simulink model "Control_try_final_2020b"  (R2020b)
settings: Solver=VariableStepAuto  StartTime=0.0  StopTime=inf  RelTol=1e-3
undefined symbols (not defined in the file or in its folder): DiscIntNeverNeededParam
libraries: mobileRoboticsLib x25
(part 4 of 7)

== system Control_try_final_2020b/Team_1_behaviour/T1R2 (attacker 1)/Team 1 Behaviour1/Subsystem1 ==
  Action Port : Inport
  In2 : Inport  Port=2
  Action Port1 : Inport  Port=3
  Constant1 : Constant  Value=5.5
  If Action Subsystem : Subsystem  TreatAsAtomicUnit=on
  If Action Subsystem1 : Subsystem  TreatAsAtomicUnit=on
  Merge : Merge
  Bx : Outport
  wires:
  Constant1/1 -> If Action Subsystem/1(In1)
  If Action Subsystem/1(reset_pos) -> Merge/1
  Action Port1/1 -> If Action Subsystem1/Action
  If Action Subsystem1/1(reset_pos) -> Merge/2
  In2/1 -> If Action Subsystem1/1(In1)
  Merge/1 -> Bx/1
  Action Port/1 -> If Action Subsystem/Action

== system Control_try_final_2020b/Team_1_behaviour/T1R2 (attacker 1)/Team 1 Behaviour1/kick_direction1 ==
  In1 : Inport
  kick : Inport  Port=2
  dF : Inport  Port=3
  Angle Finder1 : Subsystem
  Chart1 : Stateflow chart  TreatAsAtomicUnit=on
  Chart2 : Stateflow chart  TreatAsAtomicUnit=on
  Constant2 : Constant
  Cos : Trigonometry  Operator=cos
  Demux2 : Demux  Outputs=2
  Product : Product  Inputs=3
  Product1 : Product  Inputs=3
  Sin : Trigonometry
  Vector Concatenate : Concatenate  NumInputs=4
  XYZK : Outport
  wires:
  Demux2/2 -> Chart2/1(y)
  Demux2/1 -> Chart1/1(x)
  In1/1 -> Angle Finder1/1(In1), Demux2/1
  Chart1/1(Vx) -> Product/2
  Cos/1 -> Product/3
  Angle Finder1/1(angle) -> Cos/1, Sin/1
  dF/1 -> Product/1, Product1/3
  Chart2/1(Vy) -> Product1/2
  Sin/1 -> Product1/1
  Product/1 -> Vector Concatenate/1
  Product1/1 -> Vector Concatenate/2
  Constant2/1 -> Vector Concatenate/3
  kick/1 -> Vector Concatenate/4
  Vector Concatenate/1 -> XYZK/1

== system Control_try_final_2020b/Team_1_behaviour/T1R2 (attacker 1)/Team 1 Behaviour1/min_Distance_Finder ==
  R_2_sen : Inport
  R_2_loc : Inport  Port=2
  R_1_loc : Inport  Port=3
  R_3_loc : Inport  Port=4
  R_4_loc : Inport  Port=5
  Display : Display
  Display1 : Display
  Display2 : Display
  Distance1 : Subsystem
  Distance2 : Subsystem
  MATLAB Function : MATLAB Function  TreatAsAtomicUnit=on
  Min : MinMax  Inputs=2
  Min1 : MinMax  Inputs=3
  R2_O_dist_val : Subsystem
  R3_O_dist_val : Subsystem
  R4_O_dist_val : Subsystem
  zero_padding : MATLAB Function  TreatAsAtomicUnit=on
  nearest_team : Outport
  nearest_opponent : Outport  Port=2
  nearest_team_idx : Outport  Port=3
  wires:
  R_1_loc/1 -> R2_O_dist_val/2(R_2_loc)
  R_2_loc/1 -> R4_O_dist_val/1(R_1_loc), R3_O_dist_val/1(R_1_loc), R2_O_dist_val/1(R_1_loc), Distance2/1(R_1_loc), Distance1/1(R_1_loc)
  R_3_loc/1 -> R3_O_dist_val/2(R_2_loc), Distance1/2(R_3_loc)
  R_4_loc/1 -> R4_O_dist_val/2(R_2_loc), Distance2/2(R_4_loc)
  R_2_sen/1 -> zero_padding/1(u)
  zero_padding/1(y) -> R3_O_dist_val/3(sen_1_val), R4_O_dist_val/3(sen_1_val), R2_O_dist_val/3(sen_1_val)
  R2_O_dist_val/1(y) -> Min1/1, Display/1
  R3_O_dist_val/1(y) -> Min1/2, Display1/1
  R4_O_dist_val/1(y) -> Min1/3, Display2/1
  Min/1 -> MATLAB Function/1(min), nearest_team/1
  Min1/1 -> nearest_opponent/1
  Distance1/1(R1_R3_dis) -> MATLAB Function/2(rob3), Min/1
  Distance2/1(R1_R4_dis) -> Min/2
  MATLAB Function/1(y) -> nearest_team_idx/1

== system Control_try_final_2020b/Team_1_behaviour/T1R3 (Defender 2)/Team 1 Behaviour1/Angle Finder1 ==
  In1 : Inport
  Abs : Abs
  Atan : Trigonometry  Operator=atan
  Demux : Demux  Outputs=2
  Divide : Product  Inputs=/*
  angle : Outport
  wires:
  Divide/1 -> Atan/1
  Demux/2 -> Divide/2
  Demux/1 -> Divide/1
  Atan/1 -> Abs/1
  Abs/1 -> angle/1
  In1/1 -> Demux/1

== system Control_try_final_2020b/Team_1_behaviour/T1R3 (Defender 2)/Team 1 Behaviour1/Proximity_Finder_Ball1 ==
  In1 : Inport
  Demux : Demux  Outputs=2
  Sqrt : Sqrt  SaturateOnIntegerOverflow=on
  Square : Math  Operator=square  SaturateOnIntegerOverflow=on
  Square1 : Math  Operator=square  SaturateOnIntegerOverflow=on
  Sum : Sum
  DBR : Outport
  wires:
  In1/1 -> Demux/1
  Demux/1 -> Square/1
  Demux/2 -> Square1/1
  Square1/1 -> Sum/2
  Square/1 -> Sum/1
  Sum/1 -> Sqrt/1
  Sqrt/1 -> DBR/1

== system Control_try_final_2020b/Team_1_behaviour/T1R3 (Defender 2)/Team 1 Behaviour1/Proximity_Finder_Ball2 ==
  In1 : Inport
  Demux : Demux  Outputs=2
  Sqrt : Sqrt  SaturateOnIntegerOverflow=on
  Square : Math  Operator=square  SaturateOnIntegerOverflow=on
  Square1 : Math  Operator=square  SaturateOnIntegerOverflow=on
  Sum : Sum
  DBR : Outport
  wires:
  Sqrt/1 -> DBR/1
  Sum/1 -> Sqrt/1
  Square/1 -> Sum/1
  Square1/1 -> Sum/2
  Demux/2 -> Square1/1
  Demux/1 -> Square/1
  In1/1 -> Demux/1

== system Control_try_final_2020b/Team_1_behaviour/T1R3 (Defender 2)/Team 1 Behaviour1/Simulink Function ==
  f : TriggerPort  TriggerType=function-call  IsSimulinkFunction=on  FunctionName=f  FunctionVisibility=scoped  VariantControl=(inherit)
  Demux : Demux  Outputs=2
  Sqrt : Sqrt  SaturateOnIntegerOverflow=on
  Square : Math  Operator=square  SaturateOnIntegerOverflow=on
  Square1 : Math  Operator=square  SaturateOnIntegerOverflow=on
  Sum : Sum
  u : ArgIn  DisableCoverage=on  PortDimensions=[1 2]  ArgumentName=u
  y : ArgOut  DisableCoverage=on  ArgumentName=y
  wires:
  u/1 -> Demux/1
  Square/1 -> Sum/1
  Sum/1 -> Sqrt/1
  Sqrt/1 -> y/1
  Square1/1 -> Sum/2
  Demux/1 -> Square/1
  Demux/2 -> Square1/1

== system Control_try_final_2020b/Team_1_behaviour/T1R3 (Defender 2)/Team 1 Behaviour1/Subsystem1 ==
  Action Port : Inport
  In2 : Inport  Port=2
  Action Port1 : Inport  Port=3
  Constant1 : Constant  Value=3.5
  If Action Subsystem : Subsystem  TreatAsAtomicUnit=on
  If Action Subsystem1 : Subsystem  TreatAsAtomicUnit=on
  Merge : Merge
  Bx : Outport
  wires:
  Constant1/1 -> If Action Subsystem/1(In1)
  If Action Subsystem/1(reset_pos) -> Merge/1
  Action Port1/1 -> If Action Subsystem1/Action
  If Action Subsystem1/1(reset_pos) -> Merge/2
  In2/1 -> If Action Subsystem1/1(In1)
  Merge/1 -> Bx/1
  Action Port/1 -> If Action Subsystem/Action

== system Control_try_final_2020b/Team_1_behaviour/T1R3 (Defender 2)/Team 1 Behaviour1/Subsystem2 ==
  Action Port : Inport
  In2 : Inport  Port=2
  Action Port1 : Inport  Port=3
  Constant1 : Constant  Value=5.5
  If Action Subsystem : Subsystem  TreatAsAtomicUnit=on
  If Action Subsystem1 : Subsystem  TreatAsAtomicUnit=on
  Merge : Merge
  By : Outport
  wires:
  Action Port/1 -> If Action Subsystem/Action
  Merge/1 -> By/1
  In2/1 -> If Action Subsystem1/1(In1)
  If Action Subsystem1/1(reset_pos) -> Merge/2
  Action Port1/1 -> If Action Subsystem1/Action
  If Action Subsystem/1(reset_pos) -> Merge/1
  Constant1/1 -> If Action Subsystem/1(In1)

== system Control_try_final_2020b/Team_1_behaviour/T1R3 (Defender 2)/Team 1 Behaviour1/kick_direction1 ==
  In1 : Inport
  kick : Inport  Port=2
  dF : Inport  Port=3
  Angle Finder1 : Subsystem
  Chart1 : Stateflow chart  TreatAsAtomicUnit=on
  Chart2 : Stateflow chart  TreatAsAtomicUnit=on
  Constant2 : Constant
  Cos : Trigonometry  Operator=cos
  Demux2 : Demux  Outputs=2
  Product : Product  Inputs=3
  Product1 : Product  Inputs=3
  Sin : Trigonometry
  Vector Concatenate : Concatenate  NumInputs=4
  XYZK : Outport
  wires:
  Demux2/2 -> Chart2/1(y)
  Demux2/1 -> Chart1/1(x)
  In1/1 -> Angle Finder1/1(In1), Demux2/1
  Chart1/1(Vx) -> Product/2
  Cos/1 -> Product/3
  Angle Finder1/1(angle) -> Cos/1, Sin/1
  dF/1 -> Product/1, Product1/3
  Chart2/1(Vy) -> Product1/2
  Sin/1 -> Product1/1
  Product/1 -> Vector Concatenate/1
  Product1/1 -> Vector Concatenate/2
  Constant2/1 -> Vector Concatenate/3
  kick/1 -> Vector Concatenate/4
  Vector Concatenate/1 -> XYZK/1

== system Control_try_final_2020b/Team_1_behaviour/T1R3 (Defender 2)/Team 1 Behaviour1/min_Distance_Finder ==
  R_2_sen : Inport
  R_2_loc : Inport  Port=2
  R_1_loc : Inport  Port=3
  R_3_loc : Inport  Port=4
  R_4_loc : Inport  Port=5
  Display : Display
  Display1 : Display
  Display2 : Display
  Distance1 : Subsystem
  Distance2 : Subsystem
  MATLAB Function : MATLAB Function  TreatAsAtomicUnit=on
  Min : MinMax  Inputs=2
  Min1 : MinMax  Inputs=3
  R2_O_dist_val : Subsystem
  R3_O_dist_val : Subsystem
  R4_O_dist_val : Subsystem
  zero_padding : MATLAB Function  TreatAsAtomicUnit=on
  nearest_team : Outport
  nearest_opponent : Outport  Port=2
  nearest_team_idx : Outport  Port=3
  wires:
  R_1_loc/1 -> R2_O_dist_val/2(R_2_loc)
  R_2_loc/1 -> R4_O_dist_val/1(R_1_loc), R3_O_dist_val/1(R_1_loc), R2_O_dist_val/1(R_1_loc), Distance2/1(R_1_loc), Distance1/1(R_1_loc)
  R_3_loc/1 -> R3_O_dist_val/2(R_2_loc), Distance1/2(R_3_loc)
  R_4_loc/1 -> R4_O_dist_val/2(R_2_loc), Distance2/2(R_4_loc)
  R_2_sen/1 -> zero_padding/1(u)
  zero_padding/1(y) -> R3_O_dist_val/3(sen_1_val), R4_O_dist_val/3(sen_1_val), R2_O_dist_val/3(sen_1_val)
  R2_O_dist_val/1(y) -> Min1/1, Display/1
  R3_O_dist_val/1(y) -> Min1/2, Display1/1
  R4_O_dist_val/1(y) -> Min1/3, Display2/1
  Min/1 -> MATLAB Function/1(min), nearest_team/1
  Min1/1 -> nearest_opponent/1
  Distance1/1(R1_R3_dis) -> MATLAB Function/2(rob3), Min/1
  Distance2/1(R1_R4_dis) -> Min/2
  MATLAB Function/1(y) -> nearest_team_idx/1

== system Control_try_final_2020b/Team_1_behaviour/T1R3 (defender 1)/Team 1 Behaviour/Angle Finder ==
  In1 : Inport
  Abs : Abs
  Atan : Trigonometry  Operator=atan
  Demux : Demux  Outputs=2
  Divide : Product  Inputs=/*
  angle : Outport
  wires:
  Divide/1 -> Atan/1
  Demux/2 -> Divide/2
  Demux/1 -> Divide/1
  Atan/1 -> Abs/1
  Abs/1 -> angle/1
  In1/1 -> Demux/1

== system Control_try_final_2020b/Team_1_behaviour/T1R3 (defender 1)/Team 1 Behaviour/Proximity_Finder_Ball ==
  In1 : Inport
  Demux : Demux  Outputs=2
  Sqrt : Sqrt  SaturateOnIntegerOverflow=on
  Square : Math  Operator=square  SaturateOnIntegerOverflow=on
  Square1 : Math  Operator=square  SaturateOnIntegerOverflow=on
  Sum : Sum
  DBR : Outport
  wires:
  In1/1 -> Demux/1
  Demux/1 -> Square/1
  Demux/2 -> Square1/1
  Square1/1 -> Sum/2
  Square/1 -> Sum/1
  Sum/1 -> Sqrt/1
  Sqrt/1 -> DBR/1

== system Control_try_final_2020b/Team_1_behaviour/T1R3 (defender 1)/Team 1 Behaviour/kick_direction ==
  In1 : Inport
  kick : Inport  Port=2
  Angle Finder1 : Subsystem
  Chart1 : Stateflow chart  TreatAsAtomicUnit=on
  Chart2 : Stateflow chart  TreatAsAtomicUnit=on
  Constant : Constant  Value=2.5
  Constant1 : Constant  Value=2.5
  Constant2 : Constant
  Cos : Trigonometry  Operator=cos
  Demux2 : Demux  Outputs=2
  Product : Product  Inputs=3
  Product1 : Product  Inputs=3
  Sin : Trigonometry
  Vector Concatenate : Concatenate  NumInputs=4
  Out1 : Outport
  wires:
  Demux2/2 -> Chart2/1(y)
  Demux2/1 -> Chart1/1(x)
  In1/1 -> Angle Finder1/1(In1), Demux2/1
  Chart1/1(Vx) -> Product/2
  Cos/1 -> Product/3
  Angle Finder1/1(angle) -> Cos/1, Sin/1
  Constant/1 -> Product/1
  Constant1/1 -> Product1/3
  Chart2/1(Vy) -> Product1/2
  Sin/1 -> Product1/1
  Product/1 -> Vector Concatenate/1
  Product1/1 -> Vector Concatenate/2
  Constant2/1 -> Vector Concatenate/3
  kick/1 -> Vector Concatenate/4
  Vector Concatenate/1 -> Out1/1

== system Control_try_final_2020b/Team_1_behaviour/T1R3 (defender 1)/Team 1 Behaviour1/Angle Finder1 ==
  In1 : Inport
  Abs : Abs
  Atan : Trigonometry  Operator=atan
  Demux : Demux  Outputs=2
  Divide : Product  Inputs=/*
  angle : Outport
  wires:
  Divide/1 -> Atan/1
  Demux/2 -> Divide/2
  Demux/1 -> Divide/1
  Atan/1 -> Abs/1
  Abs/1 -> angle/1
  In1/1 -> Demux/1

== system Control_try_final_2020b/Team_1_behaviour/T1R3 (defender 1)/Team 1 Behaviour1/Proximity_Finder_Ball1 ==
  In1 : Inport
  Demux : Demux  Outputs=2
  Sqrt : Sqrt  SaturateOnIntegerOverflow=on
  Square : Math  Operator=square  SaturateOnIntegerOverflow=on
  Square1 : Math  Operator=square  SaturateOnIntegerOverflow=on
  Sum : Sum
  DBR : Outport
  wires:
  In1/1 -> Demux/1
  Demux/1 -> Square/1
  Demux/2 -> Square1/1
  Square1/1 -> Sum/2
  Square/1 -> Sum/1
  Sum/1 -> Sqrt/1
  Sqrt/1 -> DBR/1

== system Control_try_final_2020b/Team_1_behaviour/T1R3 (defender 1)/Team 1 Behaviour1/Proximity_Finder_Ball2 ==
  In1 : Inport
  Demux : Demux  Outputs=2
  Sqrt : Sqrt  SaturateOnIntegerOverflow=on
  Square : Math  Operator=square  SaturateOnIntegerOverflow=on
  Square1 : Math  Operator=square  SaturateOnIntegerOverflow=on
  Sum : Sum
  DBR : Outport
  wires:
  Sqrt/1 -> DBR/1
  Sum/1 -> Sqrt/1
  Square/1 -> Sum/1
  Square1/1 -> Sum/2
  Demux/2 -> Square1/1
  Demux/1 -> Square/1
  In1/1 -> Demux/1

== system Control_try_final_2020b/Team_1_behaviour/T1R3 (defender 1)/Team 1 Behaviour1/Simulink Function ==
  f : TriggerPort  TriggerType=function-call  IsSimulinkFunction=on  FunctionName=f  FunctionVisibility=scoped  VariantControl=(inherit)
  Demux : Demux  Outputs=2
  Sqrt : Sqrt  SaturateOnIntegerOverflow=on
  Square : Math  Operator=square  SaturateOnIntegerOverflow=on
  Square1 : Math  Operator=square  SaturateOnIntegerOverflow=on
  Sum : Sum
  u : ArgIn  DisableCoverage=on  PortDimensions=[1 2]  ArgumentName=u
  y : ArgOut  DisableCoverage=on  ArgumentName=y
  wires:
  u/1 -> Demux/1
  Square/1 -> Sum/1
  Sum/1 -> Sqrt/1
  Sqrt/1 -> y/1
  Square1/1 -> Sum/2
  Demux/1 -> Square/1
  Demux/2 -> Square1/1

== system Control_try_final_2020b/Team_1_behaviour/T1R3 (defender 1)/Team 1 Behaviour1/Subsystem1 ==
  Action Port : Inport
  In2 : Inport  Port=2
  Action Port1 : Inport  Port=3
  Constant1 : Constant  Value=3.5
  If Action Subsystem : Subsystem  TreatAsAtomicUnit=on
  If Action Subsystem1 : Subsystem  TreatAsAtomicUnit=on
  Merge : Merge
  Bx : Outport
  wires:
  Constant1/1 -> If Action Subsystem/1(In1)
  If Action Subsystem/1(reset_pos) -> Merge/1
  Action Port1/1 -> If Action Subsystem1/Action
  If Action Subsystem1/1(reset_pos) -> Merge/2
  In2/1 -> If Action Subsystem1/1(In1)
  Merge/1 -> Bx/1
  Action Port/1 -> If Action Subsystem/Action

== system Control_try_final_2020b/Team_1_behaviour/T1R3 (defender 1)/Team 1 Behaviour1/Subsystem2 ==
  Action Port : Inport
  In2 : Inport  Port=2
  Action Port1 : Inport  Port=3
  Constant1 : Constant  Value=2.5
  If Action Subsystem : Subsystem  TreatAsAtomicUnit=on
  If Action Subsystem1 : Subsystem  TreatAsAtomicUnit=on
  Merge : Merge
  By : Outport
  wires:
  Action Port/1 -> If Action Subsystem/Action
  Merge/1 -> By/1
  In2/1 -> If Action Subsystem1/1(In1)
  If Action Subsystem1/1(reset_pos) -> Merge/2
  Action Port1/1 -> If Action Subsystem1/Action
  If Action Subsystem/1(reset_pos) -> Merge/1
  Constant1/1 -> If Action Subsystem/1(In1)

== system Control_try_final_2020b/Team_1_behaviour/T1R3 (defender 1)/Team 1 Behaviour1/kick_direction1 ==
  In1 : Inport
  kick : Inport  Port=2
  dF : Inport  Port=3
  Angle Finder1 : Subsystem
  Chart1 : Stateflow chart  TreatAsAtomicUnit=on
  Chart2 : Stateflow chart  TreatAsAtomicUnit=on
  Constant2 : Constant
  Cos : Trigonometry  Operator=cos
  Demux2 : Demux  Outputs=2
  Product : Product  Inputs=3
  Product1 : Product  Inputs=3
  Sin : Trigonometry
  Vector Concatenate : Concatenate  NumInputs=4
  XYZK : Outport
  wires:
  Demux2/2 -> Chart2/1(y)
  Demux2/1 -> Chart1/1(x)
  In1/1 -> Angle Finder1/1(In1), Demux2/1
  Chart1/1(Vx) -> Product/2
  Cos/1 -> Product/3
  Angle Finder1/1(angle) -> Cos/1, Sin/1
  dF/1 -> Product/1, Product1/3
  Chart2/1(Vy) -> Product1/2
  Sin/1 -> Product1/1
  Product/1 -> Vector Concatenate/1
  Product1/1 -> Vector Concatenate/2
  Constant2/1 -> Vector Concatenate/3
  kick/1 -> Vector Concatenate/4
  Vector Concatenate/1 -> XYZK/1

== system Control_try_final_2020b/Team_1_behaviour/T1R3 (defender 1)/Team 1 Behaviour1/min_Distance_Finder ==
  R_2_sen : Inport
  R_2_loc : Inport  Port=2
  R_1_loc : Inport  Port=3
  R_3_loc : Inport  Port=4
  R_4_loc : Inport  Port=5
  Display : Display
  Display1 : Display
  Display2 : Display
  Distance1 : Subsystem
  Distance2 : Subsystem
  MATLAB Function : MATLAB Function  TreatAsAtomicUnit=on
  Min : MinMax  Inputs=2
  Min1 : MinMax  Inputs=3
  R2_O_dist_val : Subsystem
  R3_O_dist_val : Subsystem
  R4_O_dist_val : Subsystem
  zero_padding : MATLAB Function  TreatAsAtomicUnit=on
  nearest_team : Outport
  nearest_opponent : Outport  Port=2
  nearest_team_idx : Outport  Port=3
  wires:
  R_1_loc/1 -> R2_O_dist_val/2(R_2_loc)
  R_2_loc/1 -> R4_O_dist_val/1(R_1_loc), R3_O_dist_val/1(R_1_loc), R2_O_dist_val/1(R_1_loc), Distance2/1(R_1_loc), Distance1/1(R_1_loc)
  R_3_loc/1 -> R3_O_dist_val/2(R_2_loc), Distance1/2(R_3_loc)
  R_4_loc/1 -> R4_O_dist_val/2(R_2_loc), Distance2/2(R_4_loc)
  R_2_sen/1 -> zero_padding/1(u)
  zero_padding/1(y) -> R3_O_dist_val/3(sen_1_val), R4_O_dist_val/3(sen_1_val), R2_O_dist_val/3(sen_1_val)
  R2_O_dist_val/1(y) -> Min1/1, Display/1
  R3_O_dist_val/1(y) -> Min1/2, Display1/1
  R4_O_dist_val/1(y) -> Min1/3, Display2/1
  Min/1 -> MATLAB Function/1(min), nearest_team/1
  Min1/1 -> nearest_opponent/1
  Distance1/1(R1_R3_dis) -> MATLAB Function/2(rob3), Min/1
  Distance2/1(R1_R4_dis) -> Min/2
  MATLAB Function/1(y) -> nearest_team_idx/1

== system Control_try_final_2020b/Team_2_Behaviour/T2_R1(Goal_Keeper)/min_Distance_Finder/Distance ==
  R_1_loc : Inport
  R_2_loc : Inport  Port=2
  Demux : Demux  Outputs=3
  Demux1 : Demux  Outputs=3
  Square : Math  Operator=square  SaturateOnIntegerOverflow=on
  Square Root : Sqrt  SaturateOnIntegerOverflow=on
  Square1 : Math  Operator=square  SaturateOnIntegerOverflow=on
  Sum : Sum  Inputs=|+-
  Sum1 : Sum  Inputs=|+-
  Sum2 : Sum  Inputs=|++
  R1_R2_dis : Outport
  wires:
  Square1/1 -> Sum2/2
  Demux/2 -> Sum1/1
  Sum2/1 -> Square Root/1
  Square/1 -> Sum2/1
  Demux/1 -> Sum/1
  Sum1/1 -> Square1/1
  Demux1/2 -> Sum1/2
  Sum/1 -> Square/1
  Demux1/1 -> Sum/2
  R_1_loc/1 -> Demux/1
  R_2_loc/1 -> Demux1/1
  Square Root/1 -> R1_R2_dis/1

== system Control_try_final_2020b/Team_2_Behaviour/T2_R1(Goal_Keeper)/min_Distance_Finder/Distance1 ==
  R_1_loc : Inport
  R_3_loc : Inport  Port=2
  Demux : Demux  Outputs=3
  Demux1 : Demux  Outputs=3
  Square : Math  Operator=square  SaturateOnIntegerOverflow=on
  Square Root : Sqrt  SaturateOnIntegerOverflow=on
  Square1 : Math  Operator=square  SaturateOnIntegerOverflow=on
  Sum : Sum  Inputs=|+-
  Sum1 : Sum  Inputs=|+-
  Sum2 : Sum  Inputs=|++
  R1_R3_dis : Outport
  wires:
  Square1/1 -> Sum2/2
  Demux/2 -> Sum1/1
  Sum2/1 -> Square Root/1
  Square/1 -> Sum2/1
  Demux/1 -> Sum/1
  Sum1/1 -> Square1/1
  Demux1/2 -> Sum1/2
  Sum/1 -> Square/1
  Demux1/1 -> Sum/2
  R_1_loc/1 -> Demux/1
  R_3_loc/1 -> Demux1/1
  Square Root/1 -> R1_R3_dis/1

== system Control_try_final_2020b/Team_2_Behaviour/T2_R1(Goal_Keeper)/min_Distance_Finder/Distance2 ==
  R_1_loc : Inport
  R_4_loc : Inport  Port=2
  Demux : Demux  Outputs=3
  Demux1 : Demux  Outputs=3
  Square : Math  Operator=square  SaturateOnIntegerOverflow=on
  Square Root : Sqrt  SaturateOnIntegerOverflow=on
  Square1 : Math  Operator=square  SaturateOnIntegerOverflow=on
  Sum : Sum  Inputs=|+-
  Sum1 : Sum  Inputs=|+-
  Sum2 : Sum  Inputs=|++
  R1_R4_dis : Outport
  wires:
  Square1/1 -> Sum2/2
  Demux/2 -> Sum1/1
  Sum2/1 -> Square Root/1
  Square/1 -> Sum2/1
  Demux/1 -> Sum/1
  Sum1/1 -> Square1/1
  Demux1/2 -> Sum1/2
  Sum/1 -> Square/1
  Demux1/1 -> Sum/2
  R_1_loc/1 -> Demux/1
  R_4_loc/1 -> Demux1/1
  Square Root/1 -> R1_R4_dis/1

== system Control_try_final_2020b/Team_2_Behaviour/T2_R1(Goal_Keeper)/min_Distance_Finder/R2_O_dist_val ==
  R_1_loc : Inport
  R_2_loc : Inport  Port=2
  sen_1_val : Inport  Port=3
  Chart : Stateflow chart  TreatAsAtomicUnit=on
  y : Outport
  wires:
  sen_1_val/1 -> Chart/2(sen_1_val)
  R_1_loc/1 -> Chart/1(R_1_loc)
  R_2_loc/1 -> Chart/3(R_2_loc)
  Chart/1(dist) -> y/1

== system Control_try_final_2020b/Team_2_Behaviour/T2_R1(Goal_Keeper)/min_Distance_Finder/R3_O_dist_val ==
  R_1_loc : Inport
  R_2_loc : Inport  Port=2
  sen_1_val : Inport  Port=3
  Chart : Stateflow chart  TreatAsAtomicUnit=on
  y : Outport
  wires:
  Chart/1(dist) -> y/1
  R_2_loc/1 -> Chart/3(R_2_loc)
  R_1_loc/1 -> Chart/1(R_1_loc)
  sen_1_val/1 -> Chart/2(sen_1_val)

== system Control_try_final_2020b/Team_2_Behaviour/T2_R1(Goal_Keeper)/min_Distance_Finder/R4_O_dist_val ==
  R_1_loc : Inport
  R_2_loc : Inport  Port=2
  sen_1_val : Inport  Port=3
  Chart : Stateflow chart  TreatAsAtomicUnit=on
  y : Outport
  wires:
  sen_1_val/1 -> Chart/2(sen_1_val)
  R_1_loc/1 -> Chart/1(R_1_loc)
  R_2_loc/1 -> Chart/3(R_2_loc)
  Chart/1(dist) -> y/1

== system Control_try_final_2020b/Team_2_Behaviour/T2_R2(defender)/Team 1 Behaviour1/Angle Finder1 ==
  In1 : Inport
  Abs : Abs
  Atan : Trigonometry  Operator=atan
  Demux : Demux  Outputs=2
  Divide : Product  Inputs=/*
  angle : Outport
  wires:
  Divide/1 -> Atan/1
  Demux/2 -> Divide/2
  Demux/1 -> Divide/1
  Atan/1 -> Abs/1
  Abs/1 -> angle/1
  In1/1 -> Demux/1

== system Control_try_final_2020b/Team_2_Behaviour/T2_R2(defender)/Team 1 Behaviour1/Proximity_Finder_Ball1 ==
  In1 : Inport
  Demux : Demux  Outputs=2
  Sqrt : Sqrt  SaturateOnIntegerOverflow=on
  Square : Math  Operator=square  SaturateOnIntegerOverflow=on
  Square1 : Math  Operator=square  SaturateOnIntegerOverflow=on
  Sum : Sum
  DBR : Outport
  wires:
  In1/1 -> Demux/1
  Demux/1 -> Square/1
  Demux/2 -> Square1/1
  Square1/1 -> Sum/2
  Square/1 -> Sum/1
  Sum/1 -> Sqrt/1
  Sqrt/1 -> DBR/1

== system Control_try_final_2020b/Team_2_Behaviour/T2_R2(defender)/Team 1 Behaviour1/Proximity_Finder_Ball2 ==
  In1 : Inport
  Demux : Demux  Outputs=2
  Sqrt : Sqrt  SaturateOnIntegerOverflow=on
  Square : Math  Operator=square  SaturateOnIntegerOverflow=on
  Square1 : Math  Operator=square  SaturateOnIntegerOverflow=on
  Sum : Sum
  DBR : Outport
  wires:
  Sqrt/1 -> DBR/1
  Sum/1 -> Sqrt/1
  Square/1 -> Sum/1
  Square1/1 -> Sum/2
  Demux/2 -> Square1/1
  Demux/1 -> Square/1
  In1/1 -> Demux/1

== system Control_try_final_2020b/Team_2_Behaviour/T2_R2(defender)/Team 1 Behaviour1/Simulink Function ==
  f : TriggerPort  TriggerType=function-call  IsSimulinkFunction=on  FunctionName=f  FunctionVisibility=scoped  VariantControl=(inherit)
  Demux : Demux  Outputs=2
  Sqrt : Sqrt  SaturateOnIntegerOverflow=on
  Square : Math  Operator=square  SaturateOnIntegerOverflow=on
  Square1 : Math  Operator=square  SaturateOnIntegerOverflow=on
  Sum : Sum
  u : ArgIn  DisableCoverage=on  PortDimensions=[1 2]  ArgumentName=u
  y : ArgOut  DisableCoverage=on  ArgumentName=y
  wires:
  u/1 -> Demux/1
  Square/1 -> Sum/1
  Sum/1 -> Sqrt/1
  Sqrt/1 -> y/1
  Square1/1 -> Sum/2
  Demux/1 -> Square/1
  Demux/2 -> Square1/1

== system Control_try_final_2020b/Team_2_Behaviour/T2_R2(defender)/Team 1 Behaviour1/Subsystem ==
  Constant5 : Constant
  Constant6 : Constant  Value=4
  IC : InitialCondition  Value=0
  If : If
  If Action Subsystem : Subsystem  TreatAsAtomicUnit=on
  If Action Subsystem1 : Subsystem  TreatAsAtomicUnit=on
  Matrix Concatenate1 : Concatenate  Mode=Multidimensional array  ConcatenateDimension=2
  Merge : Merge
  Out1 : Outport
  wires:
  [centroid] -> If Action Subsystem1/1(In1)
  [A] -> IC/1
  If/1 -> If Action Subsystem/Action
  If Action Subsystem1/1(Out1) -> Merge/2
  Matrix Concatenate1/1 -> If Action Subsystem/1(In1)
  IC/1 -> If/1
  Constant6/1 -> Matrix Concatenate1/2
  Constant5/1 -> Matrix Concatenate1/1
  If/2 -> If Action Subsystem1/Action
  If Action Subsystem/1(Out1) -> Merge/1
  Merge/1 -> Out1/1

== system Control_try_final_2020b/Team_2_Behaviour/T2_R2(defender)/Team 1 Behaviour1/Subsystem1 ==
  Action Port : Inport
  In2 : Inport  Port=2
  Action Port1 : Inport  Port=3
  Constant1 : Constant  Value=7.5
  If Action Subsystem : Subsystem  TreatAsAtomicUnit=on
  If Action Subsystem1 : Subsystem  TreatAsAtomicUnit=on
  Merge : Merge
  Out1 : Outport
  wires:
  Constant1/1 -> If Action Subsystem/1(In1)
  If Action Subsystem/1(reset_pos) -> Merge/1
  Action Port1/1 -> If Action Subsystem1/Action
  If Action Subsystem1/1(reset_pos) -> Merge/2
  In2/1 -> If Action Subsystem1/1(In1)
  Merge/1 -> Out1/1
  Action Port/1 -> If Action Subsystem/Action

== system Control_try_final_2020b/Team_2_Behaviour/T2_R2(defender)/Team 1 Behaviour1/Subsystem2 ==
  Action Port : Inport
  In2 : Inport  Port=2
  Action Port1 : Inport  Port=3
  Constant1 : Constant  Value=2.5
  If Action Subsystem : Subsystem  TreatAsAtomicUnit=on
  If Action Subsystem1 : Subsystem  TreatAsAtomicUnit=on
  Merge : Merge
  By : Outport
  wires:
  Action Port/1 -> If Action Subsystem/Action
  Merge/1 -> By/1
  In2/1 -> If Action Subsystem1/1(In1)
  If Action Subsystem1/1(reset_pos) -> Merge/2
  Action Port1/1 -> If Action Subsystem1/Action
  If Action Subsystem/1(reset_pos) -> Merge/1
  Constant1/1 -> If Action Subsystem/1(In1)

== system Control_try_final_2020b/Team_2_Behaviour/T2_R2(defender)/Team 1 Behaviour1/kick_direction1 ==
  In1 : Inport
  kick : Inport  Port=2
  dF : Inport  Port=3
  Angle Finder1 : Subsystem
  Chart1 : Stateflow chart  TreatAsAtomicUnit=on
  Chart2 : Stateflow chart  TreatAsAtomicUnit=on
  Constant2 : Constant
  Cos : Trigonometry  Operator=cos
  Demux2 : Demux  Outputs=2
  Product : Product  Inputs=3
  Product1 : Product  Inputs=3
  Sin : Trigonometry
  Vector Concatenate : Concatenate  NumInputs=4
  XYZK : Outport
  wires:
  Demux2/2 -> Chart2/1(y)
  Demux2/1 -> Chart1/1(x)
  In1/1 -> Angle Finder1/1(In1), Demux2/1
  Chart1/1(Vx) -> Product/2
  Cos/1 -> Product/3
  Angle Finder1/1(angle) -> Cos/1, Sin/1
  dF/1 -> Product/1, Product1/3
  Chart2/1(Vy) -> Product1/2
  Sin/1 -> Product1/1
  Product/1 -> Vector Concatenate/1
  Product1/1 -> Vector Concatenate/2
  Constant2/1 -> Vector Concatenate/3
  kick/1 -> Vector Concatenate/4
  Vector Concatenate/1 -> XYZK/1

== system Control_try_final_2020b/Team_2_Behaviour/T2_R2(defender)/Team 1 Behaviour1/min_Distance_Finder ==
  R_2_sen : Inport
  R_2_loc : Inport  Port=2
  R_1_loc : Inport  Port=3
  R_3_loc : Inport  Port=4
  R_4_loc : Inport  Port=5
  Display : Display
  Display1 : Display
  Display2 : Display
  Distance1 : Subsystem
  Distance2 : Subsystem
  MATLAB Function : MATLAB Function  TreatAsAtomicUnit=on
  Min : MinMax  Inputs=2
  Min1 : MinMax  Inputs=3
  R2_O_dist_val : Subsystem
  R3_O_dist_val : Subsystem
  R4_O_dist_val : Subsystem
  nearest robot distance : Subsystem
  zero_padding : MATLAB Function  TreatAsAtomicUnit=on
  nearest_team : Outport
  nearest_opponent : Outport  Port=2
  nearest_team_idx : Outport  Port=3
  nearest_robot : Outport  Port=4
  wires:
  R_1_loc/1 -> R2_O_dist_val/2(R_2_loc), nearest robot distance/1(R_1_loc)
  R_2_loc/1 -> R4_O_dist_val/1(R_1_loc), R3_O_dist_val/1(R_1_loc), R2_O_dist_val/1(R_1_loc), Distance2/1(R_1_loc), Distance1/1(R_1_loc)
  R_3_loc/1 -> R3_O_dist_val/2(R_2_loc), Distance1/2(R_3_loc)
  R_4_loc/1 -> R4_O_dist_val/2(R_2_loc), Distance2/2(R_4_loc)
  R_2_sen/1 -> zero_padding/1(u)
  zero_padding/1(y) -> nearest robot distance/2(sen_1_val), R3_O_dist_val/3(sen_1_val), R4_O_dist_val/3(sen_1_val), R2_O_dist_val/3(sen_1_val)
  R2_O_dist_val/1(y) -> Min1/1, Display/1
  R3_O_dist_val/1(y) -> Min1/2, Display1/1
  R4_O_dist_val/1(y) -> Min1/3, Display2/1
  Min/1 -> MATLAB Function/1(min), nearest_team/1
  Min1/1 -> nearest_opponent/1
  Distance1/1(R1_R3_dis) -> MATLAB Function/2(rob3), Min/1
  Distance2/1(R1_R4_dis) -> Min/2
  MATLAB Function/1(y) -> nearest_team_idx/1
  nearest robot distance/1(y) -> nearest_robot/1

== system Control_try_final_2020b/Team_2_Behaviour/T2_R3(Attacker 1)/Team 1 Behaviour1/Angle Finder1 ==
  In1 : Inport
  Abs : Abs
  Atan : Trigonometry  Operator=atan
  Demux : Demux  Outputs=2
  Divide : Product  Inputs=/*
  angle : Outport
  wires:
  Divide/1 -> Atan/1
  Demux/2 -> Divide/2
  Demux/1 -> Divide/1
  Atan/1 -> Abs/1
  Abs/1 -> angle/1
  In1/1 -> Demux/1

== system Control_try_final_2020b/Team_2_Behaviour/T2_R3(Attacker 1)/Team 1 Behaviour1/Proximity_Finder_Ball2 ==
  In1 : Inport
  Demux : Demux  Outputs=2
  Sqrt : Sqrt  SaturateOnIntegerOverflow=on
  Square : Math  Operator=square  SaturateOnIntegerOverflow=on
  Square1 : Math  Operator=square  SaturateOnIntegerOverflow=on
  Sum : Sum
  DBR : Outport
  wires:
  In1/1 -> Demux/1
  Demux/1 -> Square/1
  Demux/2 -> Square1/1
  Square1/1 -> Sum/2
  Square/1 -> Sum/1
  Sum/1 -> Sqrt/1
  Sqrt/1 -> DBR/1

== system Control_try_final_2020b/Team_2_Behaviour/T2_R3(Attacker 1)/Team 1 Behaviour1/Proximity_Finder_Ball3 ==
  In1 : Inport
  Demux : Demux  Outputs=2
  Sqrt : Sqrt  SaturateOnIntegerOverflow=on
  Square : Math  Operator=square  SaturateOnIntegerOverflow=on
  Square1 : Math  Operator=square  SaturateOnIntegerOverflow=on
  Sum : Sum
  DBR : Outport
  wires:
  Sqrt/1 -> DBR/1
  Sum/1 -> Sqrt/1
  Square/1 -> Sum/1
  Square1/1 -> Sum/2
  Demux/2 -> Square1/1
  Demux/1 -> Square/1
  In1/1 -> Demux/1

== system Control_try_final_2020b/Team_2_Behaviour/T2_R3(Attacker 1)/Team 1 Behaviour1/Simulink Function ==
  f : TriggerPort  TriggerType=function-call  IsSimulinkFunction=on  FunctionName=f  FunctionVisibility=scoped  VariantControl=(inherit)
  Demux : Demux  Outputs=2
  Sqrt : Sqrt  SaturateOnIntegerOverflow=on
  Square : Math  Operator=square  SaturateOnIntegerOverflow=on
  Square1 : Math  Operator=square  SaturateOnIntegerOverflow=on
  Sum : Sum
  u : ArgIn  DisableCoverage=on  PortDimensions=[1 2]  ArgumentName=u
  y : ArgOut  DisableCoverage=on  ArgumentName=y
  wires:
  u/1 -> Demux/1
  Square/1 -> Sum/1
  Sum/1 -> Sqrt/1
  Sqrt/1 -> y/1
  Square1/1 -> Sum/2
  Demux/1 -> Square/1
  Demux/2 -> Square1/1

== system Control_try_final_2020b/Team_2_Behaviour/T2_R3(Attacker 1)/Team 1 Behaviour1/Subsystem ==
  Constant5 : Constant
  Constant6 : Constant  Value=4
  IC : InitialCondition  Value=0
  If : If
  If Action Subsystem : Subsystem  TreatAsAtomicUnit=on
  If Action Subsystem1 : Subsystem  TreatAsAtomicUnit=on
  Matrix Concatenate1 : Concatenate  Mode=Multidimensional array  ConcatenateDimension=2
  Merge : Merge
  Out1 : Outport
  wires:
  [centroid] -> If Action Subsystem1/1(In1)
  [A] -> IC/1
  If/1 -> If Action Subsystem/Action
  If Action Subsystem1/1(Out1) -> Merge/2
  Matrix Concatenate1/1 -> If Action Subsystem/1(In1)
  IC/1 -> If/1
  Constant6/1 -> Matrix Concatenate1/2
  Constant5/1 -> Matrix Concatenate1/1
  If/2 -> If Action Subsystem1/Action
  If Action Subsystem/1(Out1) -> Merge/1
  Merge/1 -> Out1/1

== system Control_try_final_2020b/Team_2_Behaviour/T2_R3(Attacker 1)/Team 1 Behaviour1/Subsystem1 ==
  Action Port : Inport
  In2 : Inport  Port=2
  Action Port1 : Inport  Port=3
  Constant1 : Constant  Value=6
  If Action Subsystem : Subsystem  TreatAsAtomicUnit=on
  If Action Subsystem1 : Subsystem  TreatAsAtomicUnit=on
  Merge : Merge
  Out1 : Outport
  wires:
  Constant1/1 -> If Action Subsystem/1(In1)
  If Action Subsystem/1(reset_pos) -> Merge/1
  Action Port1/1 -> If Action Subsystem1/Action
  If Action Subsystem1/1(reset_pos) -> Merge/2
  In2/1 -> If Action Subsystem1/1(In1)
  Merge/1 -> Out1/1
  Action Port/1 -> If Action Subsystem/Action

== system Control_try_final_2020b/Team_2_Behaviour/T2_R3(Attacker 1)/Team 1 Behaviour1/kick_direction1 ==
  In1 : Inport
  kick : Inport  Port=2
  dF : Inport  Port=3
  Angle Finder1 : Subsystem
  Chart1 : Stateflow chart  TreatAsAtomicUnit=on
  Chart2 : Stateflow chart  TreatAsAtomicUnit=on
  Constant2 : Constant
  Cos : Trigonometry  Operator=cos
  Demux2 : Demux  Outputs=2
  Product : Product  Inputs=3
  Product1 : Product  Inputs=3
  Sin : Trigonometry
  Vector Concatenate : Concatenate  NumInputs=4
  XYZK : Outport
  wires:
  Demux2/2 -> Chart2/1(y)
  Demux2/1 -> Chart1/1(x)
  In1/1 -> Angle Finder1/1(In1), Demux2/1
  Chart1/1(Vx) -> Product/2
  Cos/1 -> Product/3
  Angle Finder1/1(angle) -> Cos/1, Sin/1
  dF/1 -> Product/1, Product1/3
  Chart2/1(Vy) -> Product1/2
  Sin/1 -> Product1/1
  Product/1 -> Vector Concatenate/1
  Product1/1 -> Vector Concatenate/2
  Constant2/1 -> Vector Concatenate/3
  kick/1 -> Vector Concatenate/4
  Vector Concatenate/1 -> XYZK/1

== system Control_try_final_2020b/Team_2_Behaviour/T2_R3(Attacker 1)/Team 1 Behaviour1/min_Distance_Finder1 ==
  R_2_sen : Inport
  R_2_loc : Inport  Port=2
  R_1_loc : Inport  Port=3
  R_3_loc : Inport  Port=4
  R_4_loc : Inport  Port=5
  Display : Display
  Display1 : Display
  Display2 : Display
  Distance1 : Subsystem
  Distance2 : Subsystem
  MATLAB Function : MATLAB Function  TreatAsAtomicUnit=on
  Min : MinMax  Inputs=2
  Min1 : MinMax  Inputs=3
  R2_O_dist_val : Subsystem
  R3_O_dist_val : Subsystem
  R4_O_dist_val : Subsystem
  nearest robot distance : Subsystem
  zero_padding : MATLAB Function  TreatAsAtomicUnit=on
  nearest_team : Outport
  nearest_opponent : Outport  Port=2
  nearest_team_idx : Outport  Port=3
  nearest_robot : Outport  Port=4
  wires:
  R_1_loc/1 -> R2_O_dist_val/2(R_2_loc), nearest robot distance/1(R_1_loc)
  R_2_loc/1 -> R4_O_dist_val/1(R_1_loc), R3_O_dist_val/1(R_1_loc), R2_O_dist_val/1(R_1_loc), Distance2/1(R_1_loc), Distance1/1(R_1_loc)
  R_3_loc/1 -> R3_O_dist_val/2(R_2_loc), Distance1/2(R_3_loc)
  R_4_loc/1 -> R4_O_dist_val/2(R_2_loc), Distance2/2(R_4_loc)
  R_2_sen/1 -> zero_padding/1(u)
  zero_padding/1(y) -> nearest robot distance/2(sen_1_val), R3_O_dist_val/3(sen_1_val), R4_O_dist_val/3(sen_1_val), R2_O_dist_val/3(sen_1_val)
  R2_O_dist_val/1(y) -> Min1/1, Display/1
  R3_O_dist_val/1(y) -> Min1/2, Display1/1
  R4_O_dist_val/1(y) -> Min1/3, Display2/1
  Min/1 -> MATLAB Function/1(min), nearest_team/1
  Min1/1 -> nearest_opponent/1
  Distance1/1(R1_R3_dis) -> MATLAB Function/2(rob3), Min/1
  Distance2/1(R1_R4_dis) -> Min/2
  MATLAB Function/1(y) -> nearest_team_idx/1
  nearest robot distance/1(y) -> nearest_robot/1

== system Control_try_final_2020b/Team_2_Behaviour/T3_R4(Attacker 2)/Team 1 Behaviour1/Angle Finder2 ==
  In1 : Inport
  Abs : Abs
  Atan : Trigonometry  Operator=atan
  Demux : Demux  Outputs=2
  Divide : Product  Inputs=/*
  angle : Outport
  wires:
  Divide/1 -> Atan/1
  Demux/2 -> Divide/2
  Demux/1 -> Divide/1
  Atan/1 -> Abs/1
  Abs/1 -> angle/1
  In1/1 -> Demux/1

== system Control_try_final_2020b/Team_2_Behaviour/T3_R4(Attacker 2)/Team 1 Behaviour1/Proximity_Finder_Ball3 ==
  In1 : Inport
  Demux : Demux  Outputs=2
  Sqrt : Sqrt  SaturateOnIntegerOverflow=on
  Square : Math  Operator=square  SaturateOnIntegerOverflow=on
  Square1 : Math  Operator=square  SaturateOnIntegerOverflow=on
  Sum : Sum
  DBR : Outport
  wires:
  In1/1 -> Demux/1
  Demux/1 -> Square/1
  Demux/2 -> Square1/1
  Square1/1 -> Sum/2
  Square/1 -> Sum/1
  Sum/1 -> Sqrt/1
  Sqrt/1 -> DBR/1

== system Control_try_final_2020b/Team_2_Behaviour/T3_R4(Attacker 2)/Team 1 Behaviour1/Proximity_Finder_Ball4 ==
  In1 : Inport
  Demux : Demux  Outputs=2
  Sqrt : Sqrt  SaturateOnIntegerOverflow=on
  Square : Math  Operator=square  SaturateOnIntegerOverflow=on
  Square1 : Math  Operator=square  SaturateOnIntegerOverflow=on
  Sum : Sum
  DBR : Outport
  wires:
  Sqrt/1 -> DBR/1
  Sum/1 -> Sqrt/1
  Square/1 -> Sum/1
  Square1/1 -> Sum/2
  Demux/2 -> Square1/1
  Demux/1 -> Square/1
  In1/1 -> Demux/1

== system Control_try_final_2020b/Team_2_Behaviour/T3_R4(Attacker 2)/Team 1 Behaviour1/Simulink Function1 ==
  f : TriggerPort  TriggerType=function-call  IsSimulinkFunction=on  FunctionName=f  FunctionVisibility=scoped  VariantControl=(inherit)
  Demux : Demux  Outputs=2
  Sqrt : Sqrt  SaturateOnIntegerOverflow=on
  Square : Math  Operator=square  SaturateOnIntegerOverflow=on
  Square1 : Math  Operator=square  SaturateOnIntegerOverflow=on
  Sum : Sum
  u : ArgIn  DisableCoverage=on  PortDimensions=[1 2]  ArgumentName=u
  y : ArgOut  DisableCoverage=on  ArgumentName=y
  wires:
  u/1 -> Demux/1
  Square/1 -> Sum/1
  Sum/1 -> Sqrt/1
  Sqrt/1 -> y/1
  Square1/1 -> Sum/2
  Demux/1 -> Square/1
  Demux/2 -> Square1/1

== system Control_try_final_2020b/Team_2_Behaviour/T3_R4(Attacker 2)/Team 1 Behaviour1/Subsystem3 ==
  Constant5 : Constant
  Constant6 : Constant  Value=4
  IC : InitialCondition  Value=0
  If : If
  If Action Subsystem : Subsystem  TreatAsAtomicUnit=on
  If Action Subsystem1 : Subsystem  TreatAsAtomicUnit=on
  Matrix Concatenate1 : Concatenate  Mode=Multidimensional array  ConcatenateDimension=2
  Merge : Merge
  Out1 : Outport
  wires:
  [centroid] -> If Action Subsystem1/1(In1)
  [A] -> IC/1
  If/1 -> If Action Subsystem/Action
  If Action Subsystem1/1(Out1) -> Merge/2
  Matrix Concatenate1/1 -> If Action Subsystem/1(In1)
  IC/1 -> If/1
  Constant6/1 -> Matrix Concatenate1/2
  Constant5/1 -> Matrix Concatenate1/1
  If/2 -> If Action Subsystem1/Action
  If Action Subsystem/1(Out1) -> Merge/1
  Merge/1 -> Out1/1

== system Control_try_final_2020b/Team_2_Behaviour/T3_R4(Attacker 2)/Team 1 Behaviour1/Subsystem4 ==
  Action Port : Inport
  In2 : Inport  Port=2
  Action Port1 : Inport  Port=3
  Constant1 : Constant  Value=6
  If Action Subsystem : Subsystem  TreatAsAtomicUnit=on
  If Action Subsystem1 : Subsystem  TreatAsAtomicUnit=on
  Merge : Merge
  Out1 : Outport
  wires:
  Constant1/1 -> If Action Subsystem/1(In1)
  If Action Subsystem/1(reset_pos) -> Merge/1
  Action Port1/1 -> If Action Subsystem1/Action
  If Action Subsystem1/1(reset_pos) -> Merge/2
  In2/1 -> If Action Subsystem1/1(In1)
  Merge/1 -> Out1/1
  Action Port/1 -> If Action Subsystem/Action

== system Control_try_final_2020b/Team_2_Behaviour/T3_R4(Attacker 2)/Team 1 Behaviour1/kick_direction2 ==
  In1 : Inport
  kick : Inport  Port=2
  dF : Inport  Port=3
  Angle Finder1 : Subsystem
  Chart1 : Stateflow chart  TreatAsAtomicUnit=on
  Chart2 : Stateflow chart  TreatAsAtomicUnit=on
  Constant2 : Constant
  Cos : Trigonometry  Operator=cos
  Demux2 : Demux  Outputs=2
  Product : Product  Inputs=3
  Product1 : Product  Inputs=3
  Sin : Trigonometry
  Vector Concatenate : Concatenate  NumInputs=4
  XYZK : Outport
  wires:
  Demux2/2 -> Chart2/1(y)
  Demux2/1 -> Chart1/1(x)
  In1/1 -> Angle Finder1/1(In1), Demux2/1
  Chart1/1(Vx) -> Product/2
  Cos/1 -> Product/3
  Angle Finder1/1(angle) -> Cos/1, Sin/1
  dF/1 -> Product/1, Product1/3
  Chart2/1(Vy) -> Product1/2
  Sin/1 -> Product1/1
  Product/1 -> Vector Concatenate/1
  Product1/1 -> Vector Concatenate/2
  Constant2/1 -> Vector Concatenate/3
  kick/1 -> Vector Concatenate/4
  Vector Concatenate/1 -> XYZK/1

== system Control_try_final_2020b/Team_2_Behaviour/T3_R4(Attacker 2)/Team 1 Behaviour1/min_Distance_Finder1 ==
  R_2_sen : Inport
  R_2_loc : Inport  Port=2
  R_1_loc : Inport  Port=3
  R_3_loc : Inport  Port=4
  R_4_loc : Inport  Port=5
  Display : Display
  Display1 : Display
  Display2 : Display
  Distance1 : Subsystem
  Distance2 : Subsystem
  MATLAB Function : MATLAB Function  TreatAsAtomicUnit=on
  Min : MinMax  Inputs=2
  Min1 : MinMax  Inputs=3
  R2_O_dist_val : Subsystem
  R3_O_dist_val : Subsystem
  R4_O_dist_val : Subsystem
  nearest robot distance : Subsystem
  zero_padding : MATLAB Function  TreatAsAtomicUnit=on
  nearest_team : Outport
  nearest_opponent : Outport  Port=2
  nearest_team_idx : Outport  Port=3
  nearest_robot : Outport  Port=4
  wires:
  R_1_loc/1 -> R2_O_dist_val/2(R_2_loc), nearest robot distance/1(R_1_loc)
  R_2_loc/1 -> R4_O_dist_val/1(R_1_loc), R3_O_dist_val/1(R_1_loc), R2_O_dist_val/1(R_1_loc), Distance2/1(R_1_loc), Distance1/1(R_1_loc)
  R_3_loc/1 -> R3_O_dist_val/2(R_2_loc), Distance1/2(R_3_loc)
  R_4_loc/1 -> R4_O_dist_val/2(R_2_loc), Distance2/2(R_4_loc)
  R_2_sen/1 -> zero_padding/1(u)
  zero_padding/1(y) -> nearest robot distance/2(sen_1_val), R3_O_dist_val/3(sen_1_val), R4_O_dist_val/3(sen_1_val), R2_O_dist_val/3(sen_1_val)
  R2_O_dist_val/1(y) -> Min1/1, Display/1
  R3_O_dist_val/1(y) -> Min1/2, Display1/1
  R4_O_dist_val/1(y) -> Min1/3, Display2/1
  Min/1 -> MATLAB Function/1(min), nearest_team/1
  Min1/1 -> nearest_opponent/1
  Distance1/1(R1_R3_dis) -> MATLAB Function/2(rob3), Min/1
  Distance2/1(R1_R4_dis) -> Min/2
  MATLAB Function/1(y) -> nearest_team_idx/1
  nearest robot distance/1(y) -> nearest_robot/1

== system Control_try_final_2020b/Team_1_behaviour/T1R1(Goal_Keeper)/Ball_in_D/kick_direction/Angle Finder1 ==
  In1 : Inport
  Abs : Abs
  Atan : Trigonometry  Operator=atan
  Demux : Demux  Outputs=2
  Divide : Product  Inputs=/*
  angle : Outport
  wires:
  Divide/1 -> Atan/1
  Demux/2 -> Divide/2
  Demux/1 -> Divide/1
  Atan/1 -> Abs/1
  Abs/1 -> angle/1
  In1/1 -> Demux/1

== system Control_try_final_2020b/Team_1_behaviour/T1R2 (attacker 1)/Team 1 Behaviour1/Subsystem1/If Action Subsystem ==
  In1 : Inport
  Action Port : ActionPort  ActionPortLabel=if(u1 < 5.5)
  reset_pos : Outport
  wires:
  In1/1 -> reset_pos/1

== system Control_try_final_2020b/Team_1_behaviour/T1R2 (attacker 1)/Team 1 Behaviour1/Subsystem1/If Action Subsystem1 ==
  In1 : Inport
  Action Port : ActionPort  ActionPortLabel=else
  reset_pos : Outport
  wires:
  In1/1 -> reset_pos/1

== system Control_try_final_2020b/Team_1_behaviour/T1R2 (attacker 1)/Team 1 Behaviour1/kick_direction1/Angle Finder1 ==
  In1 : Inport
  Abs : Abs
  Atan : Trigonometry  Operator=atan
  Demux : Demux  Outputs=2
  Divide : Product  Inputs=/*
  angle : Outport
  wires:
  Divide/1 -> Atan/1
  Demux/2 -> Divide/2
  Demux/1 -> Divide/1
  Atan/1 -> Abs/1
  Abs/1 -> angle/1
  In1/1 -> Demux/1

== system Control_try_final_2020b/Team_1_behaviour/T1R2 (attacker 1)/Team 1 Behaviour1/min_Distance_Finder/Distance1 ==
  R_1_loc : Inport
  R_3_loc : Inport  Port=2
  Demux : Demux  Outputs=3
  Demux1 : Demux  Outputs=3
  Square : Math  Operator=square  SaturateOnIntegerOverflow=on
  Square Root : Sqrt  SaturateOnIntegerOverflow=on
  Square1 : Math  Operator=square  SaturateOnIntegerOverflow=on
  Sum : Sum  Inputs=|+-
  Sum1 : Sum  Inputs=|+-
  Sum2 : Sum  Inputs=|++
  R1_R3_dis : Outport
  wires:
  Square1/1 -> Sum2/2
  Demux/2 -> Sum1/1
  Sum2/1 -> Square Root/1
  Square/1 -> Sum2/1
  Demux/1 -> Sum/1
  Sum1/1 -> Square1/1
  Demux1/2 -> Sum1/2
  Sum/1 -> Square/1
  Demux1/1 -> Sum/2
  R_1_loc/1 -> Demux/1
  R_3_loc/1 -> Demux1/1
  Square Root/1 -> R1_R3_dis/1

== system Control_try_final_2020b/Team_1_behaviour/T1R2 (attacker 1)/Team 1 Behaviour1/min_Distance_Finder/Distance2 ==
  R_1_loc : Inport
  R_4_loc : Inport  Port=2
  Demux : Demux  Outputs=3
  Demux1 : Demux  Outputs=3
  Square : Math  Operator=square  SaturateOnIntegerOverflow=on
  Square Root : Sqrt  SaturateOnIntegerOverflow=on
  Square1 : Math  Operator=square  SaturateOnIntegerOverflow=on
  Sum : Sum  Inputs=|+-
  Sum1 : Sum  Inputs=|+-
  Sum2 : Sum  Inputs=|++
  R1_R4_dis : Outport
  wires:
  Square1/1 -> Sum2/2
  Demux/2 -> Sum1/1
  Sum2/1 -> Square Root/1
  Square/1 -> Sum2/1
  Demux/1 -> Sum/1
  Sum1/1 -> Square1/1
  Demux1/2 -> Sum1/2
  Sum/1 -> Square/1
  Demux1/1 -> Sum/2
  R_1_loc/1 -> Demux/1
  R_4_loc/1 -> Demux1/1
  Square Root/1 -> R1_R4_dis/1

== system Control_try_final_2020b/Team_1_behaviour/T1R2 (attacker 1)/Team 1 Behaviour1/min_Distance_Finder/R2_O_dist_val ==
  R_1_loc : Inport
  R_2_loc : Inport  Port=2
  sen_1_val : Inport  Port=3
  Chart : Stateflow chart  TreatAsAtomicUnit=on
  y : Outport
  wires:
  sen_1_val/1 -> Chart/2(sen_1_val)
  R_1_loc/1 -> Chart/1(R_1_loc)
  R_2_loc/1 -> Chart/3(R_2_loc)
  Chart/1(dist) -> y/1

== system Control_try_final_2020b/Team_1_behaviour/T1R2 (attacker 1)/Team 1 Behaviour1/min_Distance_Finder/R3_O_dist_val ==
  R_1_loc : Inport
  R_2_loc : Inport  Port=2
  sen_1_val : Inport  Port=3
  Chart : Stateflow chart  TreatAsAtomicUnit=on
  y : Outport
  wires:
  Chart/1(dist) -> y/1
  R_2_loc/1 -> Chart/3(R_2_loc)
  R_1_loc/1 -> Chart/1(R_1_loc)
  sen_1_val/1 -> Chart/2(sen_1_val)

== system Control_try_final_2020b/Team_1_behaviour/T1R2 (attacker 1)/Team 1 Behaviour1/min_Distance_Finder/R4_O_dist_val ==
  R_1_loc : Inport
  R_2_loc : Inport  Port=2
  sen_1_val : Inport  Port=3
  Chart : Stateflow chart  TreatAsAtomicUnit=on
  y : Outport
  wires:
  sen_1_val/1 -> Chart/2(sen_1_val)
  R_1_loc/1 -> Chart/1(R_1_loc)
  R_2_loc/1 -> Chart/3(R_2_loc)
  Chart/1(dist) -> y/1

== system Control_try_final_2020b/Team_1_behaviour/T1R3 (Defender 2)/Team 1 Behaviour1/Subsystem1/If Action Subsystem ==
  In1 : Inport
  Action Port : ActionPort  ActionPortLabel=if(u1 > 5.5)
  reset_pos : Outport
  wires:
  In1/1 -> reset_pos/1

== system Control_try_final_2020b/Team_1_behaviour/T1R3 (Defender 2)/Team 1 Behaviour1/Subsystem1/If Action Subsystem1 ==
  In1 : Inport
  Action Port : ActionPort  ActionPortLabel=else
  reset_pos : Outport
  wires:
  In1/1 -> reset_pos/1

== system Control_try_final_2020b/Team_1_behaviour/T1R3 (Defender 2)/Team 1 Behaviour1/Subsystem2/If Action Subsystem ==
  In1 : Inport
  Action Port : ActionPort  ActionPortLabel=if(u1 > 5.5)
  reset_pos : Outport
  wires:
  In1/1 -> reset_pos/1

== system Control_try_final_2020b/Team_1_behaviour/T1R3 (Defender 2)/Team 1 Behaviour1/Subsystem2/If Action Subsystem1 ==
  In1 : Inport
  Action Port : ActionPort  ActionPortLabel=else
  reset_pos : Outport
  wires:
  In1/1 -> reset_pos/1

== system Control_try_final_2020b/Team_1_behaviour/T1R3 (Defender 2)/Team 1 Behaviour1/kick_direction1/Angle Finder1 ==
  In1 : Inport
  Abs : Abs
  Atan : Trigonometry  Operator=atan
  Demux : Demux  Outputs=2
  Divide : Product  Inputs=/*
  angle : Outport
  wires:
  Divide/1 -> Atan/1
  Demux/2 -> Divide/2
  Demux/1 -> Divide/1
  Atan/1 -> Abs/1
  Abs/1 -> angle/1
  In1/1 -> Demux/1

== system Control_try_final_2020b/Team_1_behaviour/T1R3 (Defender 2)/Team 1 Behaviour1/min_Distance_Finder/Distance1 ==
  R_1_loc : Inport
  R_3_loc : Inport  Port=2
  Demux : Demux  Outputs=3
  Demux1 : Demux  Outputs=3
  Square : Math  Operator=square  SaturateOnIntegerOverflow=on
  Square Root : Sqrt  SaturateOnIntegerOverflow=on
  Square1 : Math  Operator=square  SaturateOnIntegerOverflow=on
  Sum : Sum  Inputs=|+-
  Sum1 : Sum  Inputs=|+-
  Sum2 : Sum  Inputs=|++
  R1_R3_dis : Outport
  wires:
  Square1/1 -> Sum2/2
  Demux/2 -> Sum1/1
  Sum2/1 -> Square Root/1
  Square/1 -> Sum2/1
  Demux/1 -> Sum/1
  Sum1/1 -> Square1/1
  Demux1/2 -> Sum1/2
  Sum/1 -> Square/1
  Demux1/1 -> Sum/2
  R_1_loc/1 -> Demux/1
  R_3_loc/1 -> Demux1/1
  Square Root/1 -> R1_R3_dis/1

== system Control_try_final_2020b/Team_1_behaviour/T1R3 (Defender 2)/Team 1 Behaviour1/min_Distance_Finder/Distance2 ==
  R_1_loc : Inport
  R_4_loc : Inport  Port=2
  Demux : Demux  Outputs=3
  Demux1 : Demux  Outputs=3
  Square : Math  Operator=square  SaturateOnIntegerOverflow=on
  Square Root : Sqrt  SaturateOnIntegerOverflow=on
  Square1 : Math  Operator=square  SaturateOnIntegerOverflow=on
  Sum : Sum  Inputs=|+-
  Sum1 : Sum  Inputs=|+-
  Sum2 : Sum  Inputs=|++
  R1_R4_dis : Outport
  wires:
  Square1/1 -> Sum2/2
  Demux/2 -> Sum1/1
  Sum2/1 -> Square Root/1
  Square/1 -> Sum2/1
  Demux/1 -> Sum/1
  Sum1/1 -> Square1/1
  Demux1/2 -> Sum1/2
  Sum/1 -> Square/1
  Demux1/1 -> Sum/2
  R_1_loc/1 -> Demux/1
  R_4_loc/1 -> Demux1/1
  Square Root/1 -> R1_R4_dis/1

== system Control_try_final_2020b/Team_1_behaviour/T1R3 (Defender 2)/Team 1 Behaviour1/min_Distance_Finder/R2_O_dist_val ==
  R_1_loc : Inport
  R_2_loc : Inport  Port=2
  sen_1_val : Inport  Port=3
  Chart : Stateflow chart  TreatAsAtomicUnit=on
  y : Outport
  wires:
  sen_1_val/1 -> Chart/2(sen_1_val)
  R_1_loc/1 -> Chart/1(R_1_loc)
  R_2_loc/1 -> Chart/3(R_2_loc)
  Chart/1(dist) -> y/1

== system Control_try_final_2020b/Team_1_behaviour/T1R3 (Defender 2)/Team 1 Behaviour1/min_Distance_Finder/R3_O_dist_val ==
  R_1_loc : Inport
  R_2_loc : Inport  Port=2
  sen_1_val : Inport  Port=3
  Chart : Stateflow chart  TreatAsAtomicUnit=on
  y : Outport
  wires:
  Chart/1(dist) -> y/1
  R_2_loc/1 -> Chart/3(R_2_loc)
  R_1_loc/1 -> Chart/1(R_1_loc)
  sen_1_val/1 -> Chart/2(sen_1_val)

== system Control_try_final_2020b/Team_1_behaviour/T1R3 (Defender 2)/Team 1 Behaviour1/min_Distance_Finder/R4_O_dist_val ==
  R_1_loc : Inport
  R_2_loc : Inport  Port=2
  sen_1_val : Inport  Port=3
  Chart : Stateflow chart  TreatAsAtomicUnit=on
  y : Outport
  wires:
  sen_1_val/1 -> Chart/2(sen_1_val)
  R_1_loc/1 -> Chart/1(R_1_loc)
  R_2_loc/1 -> Chart/3(R_2_loc)
  Chart/1(dist) -> y/1

== system Control_try_final_2020b/Team_1_behaviour/T1R3 (defender 1)/Team 1 Behaviour/kick_direction/Angle Finder1 ==
  In1 : Inport
  Abs : Abs
  Atan : Trigonometry  Operator=atan
  Demux : Demux  Outputs=2
  Divide : Product  Inputs=/*
  angle : Outport
  wires:
  Divide/1 -> Atan/1
  Demux/2 -> Divide/2
  Demux/1 -> Divide/1
  Atan/1 -> Abs/1
  Abs/1 -> angle/1
  In1/1 -> Demux/1

== system Control_try_final_2020b/Team_1_behaviour/T1R3 (defender 1)/Team 1 Behaviour1/Subsystem1/If Action Subsystem ==
  In1 : Inport
  Action Port : ActionPort  ActionPortLabel=if(u1 > 5.5)
  reset_pos : Outport
  wires:
  In1/1 -> reset_pos/1

== system Control_try_final_2020b/Team_1_behaviour/T1R3 (defender 1)/Team 1 Behaviour1/Subsystem1/If Action Subsystem1 ==
  In1 : Inport
  Action Port : ActionPort  ActionPortLabel=else
  reset_pos : Outport
  wires:
  In1/1 -> reset_pos/1

== system Control_try_final_2020b/Team_1_behaviour/T1R3 (defender 1)/Team 1 Behaviour1/Subsystem2/If Action Subsystem ==
  In1 : Inport
  Action Port : ActionPort  ActionPortLabel=if(u1 > 5.5)
  reset_pos : Outport
  wires:
  In1/1 -> reset_pos/1

== system Control_try_final_2020b/Team_1_behaviour/T1R3 (defender 1)/Team 1 Behaviour1/Subsystem2/If Action Subsystem1 ==
  In1 : Inport
  Action Port : ActionPort  ActionPortLabel=else
  reset_pos : Outport
  wires:
  In1/1 -> reset_pos/1

== system Control_try_final_2020b/Team_1_behaviour/T1R3 (defender 1)/Team 1 Behaviour1/kick_direction1/Angle Finder1 ==
  In1 : Inport
  Abs : Abs
  Atan : Trigonometry  Operator=atan
  Demux : Demux  Outputs=2
  Divide : Product  Inputs=/*
  angle : Outport
  wires:
  Divide/1 -> Atan/1
  Demux/2 -> Divide/2
  Demux/1 -> Divide/1
  Atan/1 -> Abs/1
  Abs/1 -> angle/1
  In1/1 -> Demux/1
